simulink model "SimControlador"  (R2025b)
settings: Solver=VariableStepAuto  StartTime=0.0  StopTime=tfin  MaxStep=0.01  RelTol=1e-3
values from neighbouring files (symbols this model uses):
  A = max(U)    [AllModels.m]    (also in ConfigurarControl.m = 40; Danier.m; Prueba2.m = 40; PruebaSegundoorden.m)
  den = [tao 1]    [ConfigurarControl.m]    (also in Prueba2.m)
  Kc = 2.5    [ConfigurarControl.m]    (also in Prueba2.m)
  Kc_i = 0.5    [ConfigurarControl.m]    (also in Prueba2.m)
  num = Kp    (= 0.83)    [ConfigurarControl.m]    (also in Prueba2.m)
  tdead = 27.8    [ConfigurarControl.m]    (also in Prueba2.m)
  tesc = 5    [ConfigurarControl.m]    (also in Prueba2.m)
  ti = 10    [ConfigurarControl.m]    (also in Prueba2.m = 20)
settings Model: Creator=b03s217  LastModifiedBy=Nehir RT
settings SolverCC: AlgebraicLoopSolver=TrustRegion
settings DebuggingCC: UnconnectedInputMsg=warning  UnconnectedOutputMsg=warning  UnconnectedLineMsg=warning
settings ModelReferenceCC: EnableRefExpFcnMdlSchedulingChecks=on
settings RTWCC: GPUComputeCapability=3.5  DLArmComputeVersion=19.05

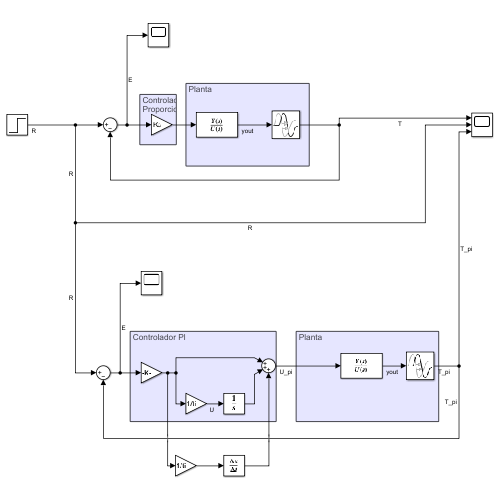
[thumbnail: Simulink's stored preview of the top-level diagram]
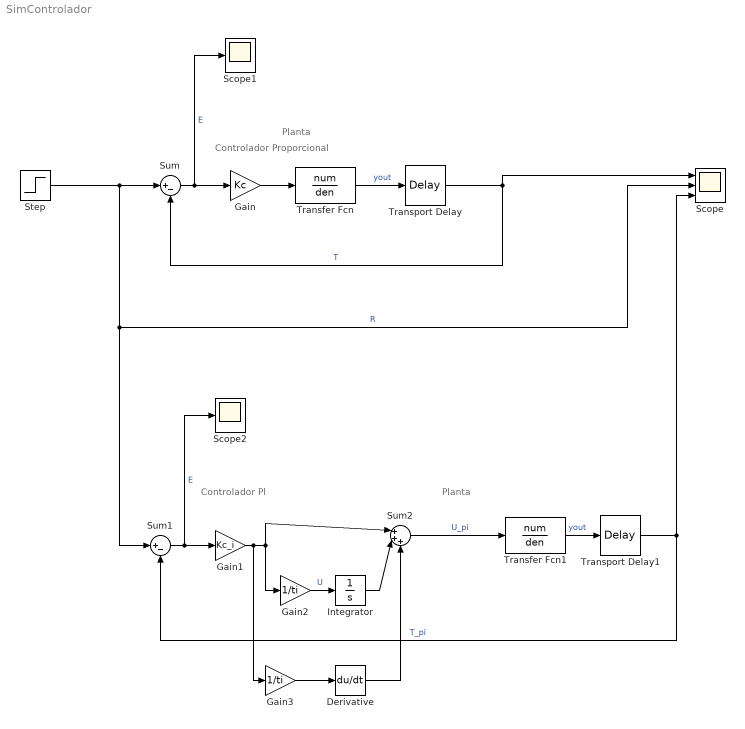
== system SimControlador ==
  note: Controlador
      | Proporcional
  note: Planta
  note: Planta
  note: Controlador Pl
  Derivative : Derivative
  Gain : Gain  Gain=Kc
  Gain1 : Gain  Gain=Kc_i
  Gain2 : Gain  Gain=1/ti
  Gain3 : Gain  Gain=1/ti
  Integrator : Integrator
  Scope : Scope  NumInputPorts=3
      settings: ActiveDisplayYMinimum=-9.23126907438003  ActiveDisplayYMaximum=67.3849650757862  DataLoggingVariableName=DatosOut
  Scope1 : Scope
      settings: ActiveDisplayYMinimum=-4.9531552004658055  ActiveDisplayYMaximum=6.9389417786363685  DataLoggingVariableName=DatosOut1
  Scope2 : Scope
      settings: ActiveDisplayYMinimum=-4.9531552004658055  ActiveDisplayYMaximum=6.9389417786363685  DataLoggingVariableName=DatosOut2
  Step : Step  Time=tesc  After=A  SampleTime=0
  Sum : Sum  Inputs=|+-
  Sum1 : Sum  Inputs=|+-
  Sum2 : Sum  Inputs=|+++
  Transfer Fcn : TransferFcn  Numerator=num  Denominator=den
  Transfer Fcn1 : TransferFcn  Numerator=num  Denominator=den
  Transport Delay : TransportDelay  DelayTime=tdead
  Transport Delay1 : TransportDelay  DelayTime=tdead
  wires:
  Transfer Fcn/1 -> Transport Delay/1  "yout"
  Transport Delay/1 -> Sum/2, Scope/1  "T"
  Step/1 -> Sum1/1, Scope/2, Sum/1  "R"
  Sum/1 -> Gain/1, Scope1/1  "E"
  Gain/1 -> Transfer Fcn/1
  Sum1/1 -> Gain1/1, Scope2/1  "E"
  Transfer Fcn1/1 -> Transport Delay1/1  "yout"
  Transport Delay1/1 -> Sum1/2, Scope/3  "T_pi"
  Gain1/1 -> Gain3/1, Sum2/1, Gain2/1
  Sum2/1 -> Transfer Fcn1/1  "U_pi"
  Gain2/1 -> Integrator/1  "U"
  Integrator/1 -> Sum2/2
  Derivative/1 -> Sum2/3
  Gain3/1 -> Derivative/1
